simulink subsystem "BEV4EM"  (R2024b)
settings: Solver=VariableStepAuto  StartTime=0.0  StopTime=10.0  RelTol=1e-3
undefined symbols (not defined in the file): PlntDriveshftDamp, PlntDriveshftStiff, PlntEM1RotDamp, PlntEM1RotInertia, PlntEM2RotDamp, PlntEM2RotInertia, PlntEM3RotDamp, PlntEM3RotInertia, PlntEM4RotDamp, PlntEM4RotInertia
libraries: autolibsharedcoupling x8
settings Model: ModifiedByFormat=The MathWorks, Inc.  Creator=The MathWorks, Inc.  LastModifiedBy=The MathWorks, Inc.
settings OptimizationCC: ReuseModelBlockBuffer=off
settings DebuggingCC: SubsystemReferenceDiagnosticForUnitTest=warning
settings RTWCC: GPUComputeCapability=3.5

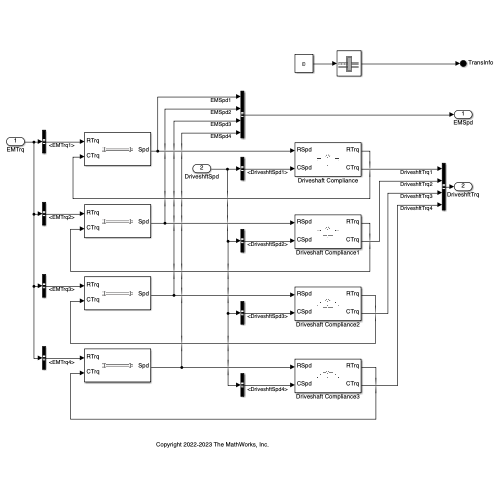
[thumbnail: Simulink's stored preview of the top-level diagram]
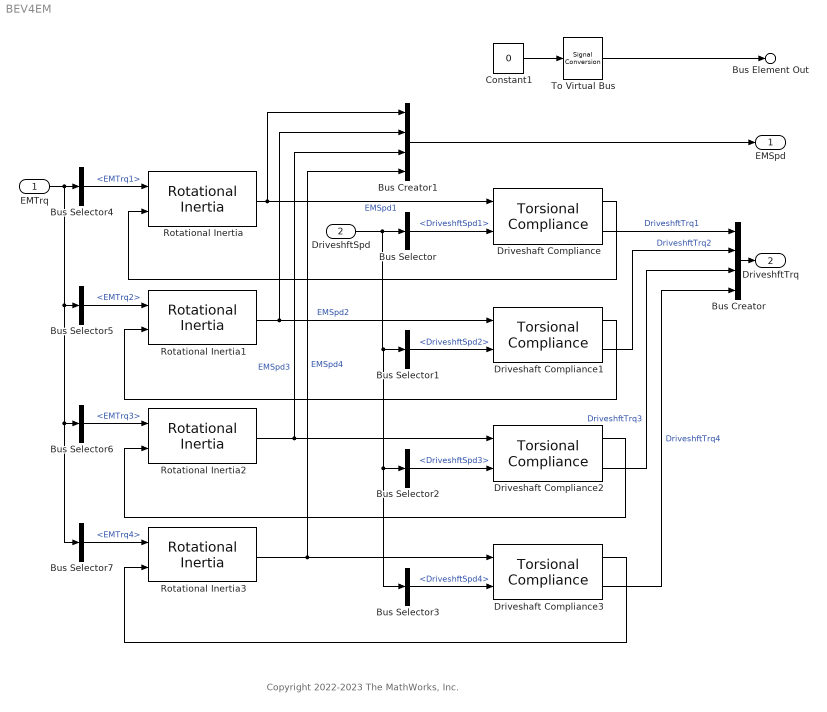
== system BEV4EM ==
  note: Copyright 2022-2023 The MathWorks, Inc.
  EMTrq : Inport
  DriveshftSpd : Inport  Port=2
  Bus Creator : BusCreator  Inputs=4
  Bus Creator1 : BusCreator  Inputs=4
  Bus Selector : BusSelector  OutputSignals=FrntDriveshftSpd.DriveshftSpd1
  Bus Selector1 : BusSelector  OutputSignals=FrntDriveshftSpd.DriveshftSpd2
  Bus Selector2 : BusSelector  OutputSignals=RearDriveshftSpd.DriveshftSpd3
  Bus Selector3 : BusSelector  OutputSignals=RearDriveshftSpd.DriveshftSpd4
  Bus Selector4 : BusSelector  OutputSignals=EMTrq1
  Bus Selector5 : BusSelector  OutputSignals=EMTrq2
  Bus Selector6 : BusSelector  OutputSignals=EMTrq3
  Bus Selector7 : BusSelector  OutputSignals=EMTrq4
  Constant1 : Constant  Value=0  OutDataTypeStr=Bus: TransInfoBUS  SampleTime=Inf
  Driveshaft Compliance{,1..3} (4 alike) : autolibsharedcoupling/Torsional Compliance  port_config=Simulink  extInfo=off  k=PlntDriveshftStiff  b=PlntDriveshftDamp  theta_o=PlntDriveshftInitDeflect  domega_o=PlntDriveshftInitVel  omega_c=PlntDriveshftDampCutoffFreq  blkID=0  aMode=1
  Rotational Inertia : autolibsharedcoupling/Rotational Inertia  port_config=Simulink  extInfo=off  externJ=off  J=PlntEM1RotInertia  b=PlntEM1RotDamp  omega_o=PlntEM1RotInitSpd  blkID=0  aMode=1
      settings: LibrarySourceBlock=autolibcoupling/Rotational Inertia
  Rotational Inertia1 : autolibsharedcoupling/Rotational Inertia  port_config=Simulink  extInfo=off  externJ=off  J=PlntEM2RotInertia  b=PlntEM2RotDamp  omega_o=PlntEM2RotInitSpd  blkID=0  aMode=1
      settings: LibrarySourceBlock=autolibcoupling/Rotational Inertia
  Rotational Inertia2 : autolibsharedcoupling/Rotational Inertia  port_config=Simulink  extInfo=off  externJ=off  J=PlntEM3RotInertia  b=PlntEM3RotDamp  omega_o=PlntEM3RotInitSpd  blkID=0  aMode=1
      settings: LibrarySourceBlock=autolibcoupling/Rotational Inertia
  Rotational Inertia3 : autolibsharedcoupling/Rotational Inertia  port_config=Simulink  extInfo=off  externJ=off  J=PlntEM4RotInertia  b=PlntEM4RotDamp  omega_o=PlntEM4RotInitSpd  blkID=0  aMode=1
      settings: LibrarySourceBlock=autolibcoupling/Rotational Inertia
  To Virtual Bus : SignalConversion  ConversionOutput=Virtual bus  OverrideOpt=off
  EMSpd : Outport  VectorParamsAs1DForOutWhenUnconnected=off  BusOutputAsStruct=on
  DriveshftTrq : Outport  Port=2  VectorParamsAs1DForOutWhenUnconnected=off
  Bus Element Out : Outport  Port=3  PortName=TransInfo
  wires:
  Bus Creator1/1 -> EMSpd/1
  Bus Selector5/1 -> Rotational Inertia1/1  "<EMTrq2>"
  Bus Creator/1 -> DriveshftTrq/1
  Driveshaft Compliance1/2 -> Bus Creator/2  "DriveshftTrq2"
  Bus Selector/1 -> Driveshaft Compliance/2  "<DriveshftSpd1>"
  Rotational Inertia1/1 -> Driveshaft Compliance1/1, Bus Creator1/2  "EMSpd2"
  Driveshaft Compliance/2 -> Bus Creator/1  "DriveshftTrq1"
  Driveshaft Compliance/1 -> Rotational Inertia/2
  Driveshaft Compliance1/1 -> Rotational Inertia1/2
  Rotational Inertia/1 -> Driveshaft Compliance/1, Bus Creator1/1  "EMSpd1"
  Bus Selector1/1 -> Driveshaft Compliance1/2  "<DriveshftSpd2>"
  Bus Selector2/1 -> Driveshaft Compliance2/2  "<DriveshftSpd3>"
  Driveshaft Compliance2/1 -> Rotational Inertia2/2
  Rotational Inertia2/1 -> Driveshaft Compliance2/1, Bus Creator1/3  "EMSpd3"
  Driveshaft Compliance2/2 -> Bus Creator/3  "DriveshftTrq3"
  Bus Selector6/1 -> Rotational Inertia2/1  "<EMTrq3>"
  Bus Selector7/1 -> Rotational Inertia3/1  "<EMTrq4>"
  Driveshaft Compliance3/2 -> Bus Creator/4  "DriveshftTrq4"
  Rotational Inertia3/1 -> Driveshaft Compliance3/1, Bus Creator1/4  "EMSpd4"
  DriveshftSpd/1 -> Bus Selector2/1, Bus Selector3/1, Bus Selector1/1, Bus Selector/1
  Driveshaft Compliance3/1 -> Rotational Inertia3/2
  Bus Selector3/1 -> Driveshaft Compliance3/2  "<DriveshftSpd4>"
  EMTrq/1 -> Bus Selector6/1, Bus Selector7/1, Bus Selector5/1, Bus Selector4/1
  Constant1/1 -> To Virtual Bus/1
  To Virtual Bus/1 -> Bus Element Out/1
  Bus Selector4/1 -> Rotational Inertia/1  "<EMTrq1>"
